simulink model "cic"  (Simulink 6.6)
settings: Solver=VariableStepDiscrete  SolverMode=SingleTasking  StartTime=0.0  StopTime=32768/12.8e6  RelTol=1e-3
PreLoadFcn:
  | load_downconverter_input
undefined symbols (not defined in the file): dfilt
libraries: xbsIndex_r4 x66, dsparch4 x3, dspsigops x2
(part 2 of 2)

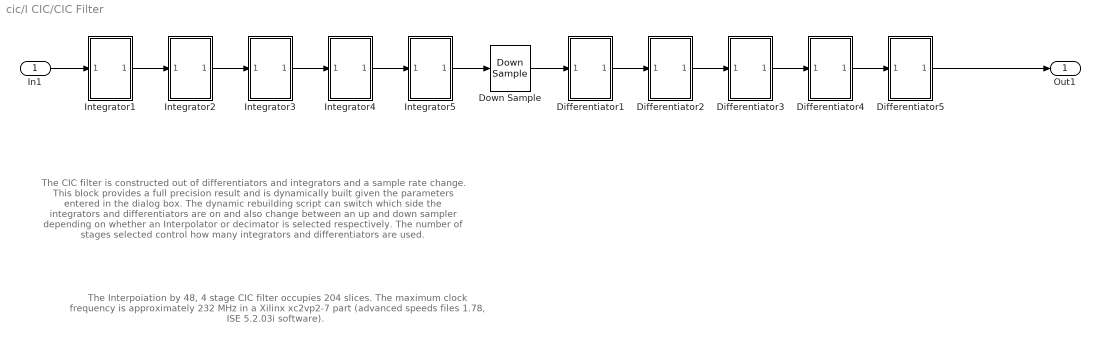
== system cic/I CIC/CIC Filter ==
  note: The Interpoiation by 48, 4 stage CIC filter occupies 204 slices.
      | The maximum clock frequency is approximately
      | 232 MHz in a Xilinx xc2vp2-7 part (advanced speeds
      | files 1.78, ISE 5.2.03i software).
  note: The CIC filter is constructed out of differentiators and integrators and
      | a sample rate change. This block provides a full precision result and is
      | dynamically built given the parameters entered in the dialog box. The
      | dynamic rebuilding script can switch which side the integrators and
      | differentiators are on and also change between an up and down sampler
      | depending on whether an Interpolator or decimator is selected respectively.
      | The number of stages selected control how many integrators and
      | differentiators are used.
  In1 : Inport
  Differentiator1 : Subsystem  mask(Differentiator Stage){m=m, output_bitwidth=ceil(stages*log2(rate_change*m) + input_bitwidth), output_binpt=input_binpt}
      mask prompts: m "Differential Delay"; output_bitwidth "Output Bit Width"; output_binpt "Output Binary Point"
      mask help: Multi-Channel Differentiator
      mask init:
      | set_param(gcb, 'LinkStatus', 'none');
  Differentiator2 : Subsystem  mask(Differentiator Stage){m=m, output_bitwidth=ceil(stages*log2(rate_change*m) + input_bitwidth), output_binpt=input_binpt}
      mask prompts: m "Differential Delay"; output_bitwidth "Output Bit Width"; output_binpt "Output Binary Point"
      mask help: Multi-Channel Differentiator
      mask init:
      | set_param(gcb, 'LinkStatus', 'none');
  Differentiator3 : Subsystem  mask(Differentiator Stage){m=m, output_bitwidth=ceil(stages*log2(rate_change*m) + input_bitwidth), output_binpt=input_binpt}
      mask prompts: m "Differential Delay"; output_bitwidth "Output Bit Width"; output_binpt "Output Binary Point"
      mask help: Multi-Channel Differentiator
      mask init:
      | set_param(gcb, 'LinkStatus', 'none');
  Differentiator4 : Subsystem  mask(Differentiator Stage){m=m, output_bitwidth=ceil(stages*log2(rate_change*m) + input_bitwidth), output_binpt=input_binpt}
      mask prompts: m "Differential Delay"; output_bitwidth "Output Bit Width"; output_binpt "Output Binary Point"
      mask help: Multi-Channel Differentiator
      mask init:
      | set_param(gcb, 'LinkStatus', 'none');
  Differentiator5 : Subsystem  mask(Differentiator Stage){m=m, output_bitwidth=ceil(stages*log2(rate_change*m) + input_bitwidth), output_binpt=input_binpt}
      mask prompts: m "Differential Delay"; output_bitwidth "Output Bit Width"; output_binpt "Output Binary Point"
      mask help: Multi-Channel Differentiator
      mask init:
      | set_param(gcb, 'LinkStatus', 'none');
  Down Sample : xbsIndex_r4/Down Sample  sample_ratio=rate_change  sample_phase=First Value of Frame  en=off  latency=1  dbl_ovrd=off  block_type=dsamp
      settings: block_version=VER_STRING_GOES_HERE
  Integrator1 : Subsystem  mask(Integrator Stage){output_bitwidth=ceil(stages*log2(rate_change*m) + input_bitwidth)}
      mask prompts: output_bitwidth "Output Bit Width"
      mask help: Multi Channel Integrator
      mask init:
      | set_param(gcb, 'LinkStatus', 'none');
      settings: CopyFcn=set_param(gcb, 'LinkStatus', 'none');
  Integrator2 : Subsystem  mask(Integrator Stage){output_bitwidth=ceil(stages*log2(rate_change*m) + input_bitwidth)}
      mask prompts: output_bitwidth "Output Bit Width"
      mask help: Multi Channel Integrator
      mask init:
      | set_param(gcb, 'LinkStatus', 'none');
      settings: CopyFcn=set_param(gcb, 'LinkStatus', 'none');
  Integrator3 : Subsystem  mask(Integrator Stage){output_bitwidth=ceil(stages*log2(rate_change*m) + input_bitwidth)}
      mask prompts: output_bitwidth "Output Bit Width"
      mask help: Multi Channel Integrator
      mask init:
      | set_param(gcb, 'LinkStatus', 'none');
      settings: CopyFcn=set_param(gcb, 'LinkStatus', 'none');
  Integrator4 : Subsystem  mask(Integrator Stage){output_bitwidth=ceil(stages*log2(rate_change*m) + input_bitwidth)}
      mask prompts: output_bitwidth "Output Bit Width"
      mask help: Multi Channel Integrator
      mask init:
      | set_param(gcb, 'LinkStatus', 'none');
      settings: CopyFcn=set_param(gcb, 'LinkStatus', 'none');
  Integrator5 : Subsystem  mask(Integrator Stage){output_bitwidth=ceil(stages*log2(rate_change*m) + input_bitwidth)}
      mask prompts: output_bitwidth "Output Bit Width"
      mask help: Multi Channel Integrator
      mask init:
      | set_param(gcb, 'LinkStatus', 'none');
      settings: CopyFcn=set_param(gcb, 'LinkStatus', 'none');
  Out1 : Outport
  wires:
  In1/1 -> Integrator1/1(In1)
  Down Sample/1 -> Differentiator1/1(In1)
  Integrator1/1(Out1) -> Integrator2/1(In1)
  Differentiator1/1(Out1) -> Differentiator2/1(In1)
  Integrator2/1(Out1) -> Integrator3/1(In1)
  Differentiator2/1(Out1) -> Differentiator3/1(In1)
  Integrator3/1(Out1) -> Integrator4/1(In1)
  Differentiator3/1(Out1) -> Differentiator4/1(In1)
  Integrator4/1(Out1) -> Integrator5/1(In1)
  Differentiator4/1(Out1) -> Differentiator5/1(In1)
  Integrator5/1(Out1) -> Down Sample/1
  Differentiator5/1(Out1) -> Out1/1

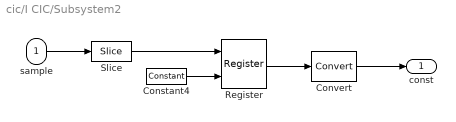
== system cic/I CIC/Subsystem2 ==
  sample : Inport
  Constant4 : xbsIndex_r4/Constant  arith_type=Boolean  const=0  n_bits=1  bin_pt=0  explicit_period=off  period=1  equ=P=C  opselect=C  inp2=PCIN>>17  opr=+  inp1=P  carry=CIN  dbl_ovrd=off  block_type=constant
      settings: block_version=VER_STRING_GOES_HERE
  Convert : xbsIndex_r4/Convert  arith_type=Boolean  n_bits=16  bin_pt=14  quantization=Truncate  overflow=Wrap  latency=0  dbl_ovrd=off  pipeline=off  block_type=convert
      settings: block_version=VER_STRING_GOES_HERE
  Register : xbsIndex_r4/Register  init=1  rst=off  en=on  dbl_ovrd=off  block_type=register
      settings: block_version=VER_STRING_GOES_HERE
  Slice : xbsIndex_r4/Slice  nbits=1  boolean_output=off  mode=Upper Bit Location + Width  bit1=0  base1=MSB of Input  bit0=0  base0=LSB of Input  dbl_ovrd=off  block_type=slice
      settings: infoedit="Extracts a given range of bits from each input sample and presents it at the output.  The output type is ordinarily unsigned with binary point at zero, but can be Boolean when the slice is one bit wide.<P><P>Hardware notes: In hardware this block costs nothing."  block_version=VER_STRING_GOES_HERE
  const : Outport
  wires:
  Constant4/1 -> Register/2
  Slice/1 -> Register/1
  sample/1 -> Slice/1
  Register/1 -> Convert/1
  Convert/1 -> const/1

== system cic/I baseband/I source ==
  Random Number2 : RandomNumber  Seed=777  SampleTime=1/100e3
  Sign2 : Signum
  Out1 : Outport
  wires:
  Random Number2/1 -> Sign2/1
  Sign2/1 -> Out1/1

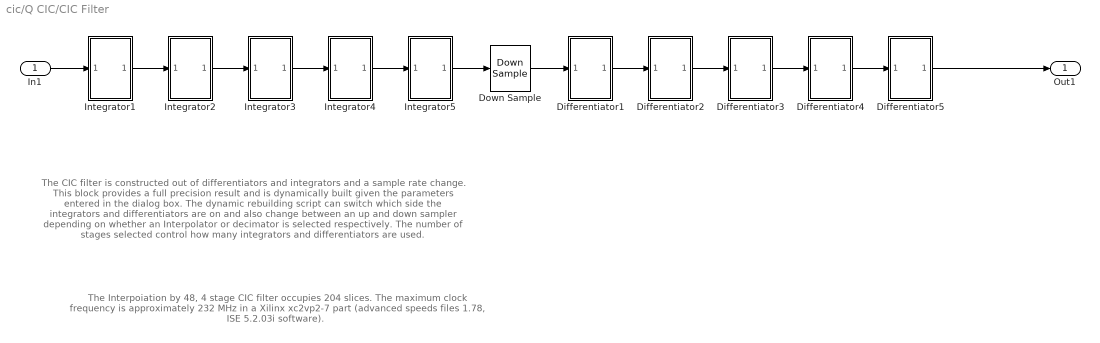
== system cic/Q CIC/CIC Filter ==
  note: The Interpoiation by 48, 4 stage CIC filter occupies 204 slices.
      | The maximum clock frequency is approximately
      | 232 MHz in a Xilinx xc2vp2-7 part (advanced speeds
      | files 1.78, ISE 5.2.03i software).
  note: The CIC filter is constructed out of differentiators and integrators and
      | a sample rate change. This block provides a full precision result and is
      | dynamically built given the parameters entered in the dialog box. The
      | dynamic rebuilding script can switch which side the integrators and
      | differentiators are on and also change between an up and down sampler
      | depending on whether an Interpolator or decimator is selected respectively.
      | The number of stages selected control how many integrators and
      | differentiators are used.
  In1 : Inport
  Differentiator1 : Subsystem  mask(Differentiator Stage){m=m, output_bitwidth=ceil(stages*log2(rate_change*m) + input_bitwidth), output_binpt=input_binpt}
      mask prompts: m "Differential Delay"; output_bitwidth "Output Bit Width"; output_binpt "Output Binary Point"
      mask help: Multi-Channel Differentiator
      mask init:
      | set_param(gcb, 'LinkStatus', 'none');
  Differentiator2 : Subsystem  mask(Differentiator Stage){m=m, output_bitwidth=ceil(stages*log2(rate_change*m) + input_bitwidth), output_binpt=input_binpt}
      mask prompts: m "Differential Delay"; output_bitwidth "Output Bit Width"; output_binpt "Output Binary Point"
      mask help: Multi-Channel Differentiator
      mask init:
      | set_param(gcb, 'LinkStatus', 'none');
  Differentiator3 : Subsystem  mask(Differentiator Stage){m=m, output_bitwidth=ceil(stages*log2(rate_change*m) + input_bitwidth), output_binpt=input_binpt}
      mask prompts: m "Differential Delay"; output_bitwidth "Output Bit Width"; output_binpt "Output Binary Point"
      mask help: Multi-Channel Differentiator
      mask init:
      | set_param(gcb, 'LinkStatus', 'none');
  Differentiator4 : Subsystem  mask(Differentiator Stage){m=m, output_bitwidth=ceil(stages*log2(rate_change*m) + input_bitwidth), output_binpt=input_binpt}
      mask prompts: m "Differential Delay"; output_bitwidth "Output Bit Width"; output_binpt "Output Binary Point"
      mask help: Multi-Channel Differentiator
      mask init:
      | set_param(gcb, 'LinkStatus', 'none');
  Differentiator5 : Subsystem  mask(Differentiator Stage){m=m, output_bitwidth=ceil(stages*log2(rate_change*m) + input_bitwidth), output_binpt=input_binpt}
      mask prompts: m "Differential Delay"; output_bitwidth "Output Bit Width"; output_binpt "Output Binary Point"
      mask help: Multi-Channel Differentiator
      mask init:
      | set_param(gcb, 'LinkStatus', 'none');
  Down Sample : xbsIndex_r4/Down Sample  sample_ratio=rate_change  sample_phase=First Value of Frame  en=off  latency=1  dbl_ovrd=off  block_type=dsamp
      settings: block_version=VER_STRING_GOES_HERE
  Integrator1 : Subsystem  mask(Integrator Stage){output_bitwidth=ceil(stages*log2(rate_change*m) + input_bitwidth)}
      mask prompts: output_bitwidth "Output Bit Width"
      mask help: Multi Channel Integrator
      mask init:
      | set_param(gcb, 'LinkStatus', 'none');
      settings: CopyFcn=set_param(gcb, 'LinkStatus', 'none');
  Integrator2 : Subsystem  mask(Integrator Stage){output_bitwidth=ceil(stages*log2(rate_change*m) + input_bitwidth)}
      mask prompts: output_bitwidth "Output Bit Width"
      mask help: Multi Channel Integrator
      mask init:
      | set_param(gcb, 'LinkStatus', 'none');
      settings: CopyFcn=set_param(gcb, 'LinkStatus', 'none');
  Integrator3 : Subsystem  mask(Integrator Stage){output_bitwidth=ceil(stages*log2(rate_change*m) + input_bitwidth)}
      mask prompts: output_bitwidth "Output Bit Width"
      mask help: Multi Channel Integrator
      mask init:
      | set_param(gcb, 'LinkStatus', 'none');
      settings: CopyFcn=set_param(gcb, 'LinkStatus', 'none');
  Integrator4 : Subsystem  mask(Integrator Stage){output_bitwidth=ceil(stages*log2(rate_change*m) + input_bitwidth)}
      mask prompts: output_bitwidth "Output Bit Width"
      mask help: Multi Channel Integrator
      mask init:
      | set_param(gcb, 'LinkStatus', 'none');
      settings: CopyFcn=set_param(gcb, 'LinkStatus', 'none');
  Integrator5 : Subsystem  mask(Integrator Stage){output_bitwidth=ceil(stages*log2(rate_change*m) + input_bitwidth)}
      mask prompts: output_bitwidth "Output Bit Width"
      mask help: Multi Channel Integrator
      mask init:
      | set_param(gcb, 'LinkStatus', 'none');
      settings: CopyFcn=set_param(gcb, 'LinkStatus', 'none');
  Out1 : Outport
  wires:
  In1/1 -> Integrator1/1(In1)
  Down Sample/1 -> Differentiator1/1(In1)
  Integrator1/1(Out1) -> Integrator2/1(In1)
  Differentiator1/1(Out1) -> Differentiator2/1(In1)
  Integrator2/1(Out1) -> Integrator3/1(In1)
  Differentiator2/1(Out1) -> Differentiator3/1(In1)
  Integrator3/1(Out1) -> Integrator4/1(In1)
  Differentiator3/1(Out1) -> Differentiator4/1(In1)
  Integrator4/1(Out1) -> Integrator5/1(In1)
  Differentiator4/1(Out1) -> Differentiator5/1(In1)
  Integrator5/1(Out1) -> Down Sample/1
  Differentiator5/1(Out1) -> Out1/1

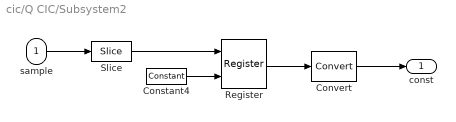
== system cic/Q CIC/Subsystem2 ==
  sample : Inport
  Constant4 : xbsIndex_r4/Constant  arith_type=Boolean  const=0  n_bits=1  bin_pt=0  explicit_period=off  period=1  equ=P=C  opselect=C  inp2=PCIN>>17  opr=+  inp1=P  carry=CIN  dbl_ovrd=off  block_type=constant
      settings: block_version=VER_STRING_GOES_HERE
  Convert : xbsIndex_r4/Convert  arith_type=Boolean  n_bits=16  bin_pt=14  quantization=Truncate  overflow=Wrap  latency=0  dbl_ovrd=off  pipeline=off  block_type=convert
      settings: block_version=VER_STRING_GOES_HERE
  Register : xbsIndex_r4/Register  init=1  rst=off  en=on  dbl_ovrd=off  block_type=register
      settings: block_version=VER_STRING_GOES_HERE
  Slice : xbsIndex_r4/Slice  nbits=1  boolean_output=off  mode=Upper Bit Location + Width  bit1=0  base1=MSB of Input  bit0=0  base0=LSB of Input  dbl_ovrd=off  block_type=slice
      settings: infoedit="Extracts a given range of bits from each input sample and presents it at the output.  The output type is ordinarily unsigned with binary point at zero, but can be Boolean when the slice is one bit wide.<P><P>Hardware notes: In hardware this block costs nothing."  block_version=VER_STRING_GOES_HERE
  const : Outport
  wires:
  Constant4/1 -> Register/2
  Slice/1 -> Register/1
  sample/1 -> Slice/1
  Register/1 -> Convert/1
  Convert/1 -> const/1

== system cic/Q baseband/Q source ==
  Random Number1 : RandomNumber  Seed=99  SampleTime=1/100e3
  Sign1 : Signum
  Out1 : Outport
  wires:
  Random Number1/1 -> Sign1/1
  Sign1/1 -> Out1/1

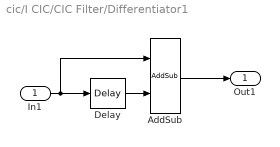
== system cic/I CIC/CIC Filter/Differentiator1 ==
  In1 : Inport
  AddSub : xbsIndex_r4/AddSub  mode=Subtraction  use_carryin=off  use_carryout=off  en=off  latency=1  precision=User Defined  arith_type="Signed  (2's comp)"  n_bits=output_bitwidth  bin_pt=output_binpt  quantization=Truncate  overflow=Wrap  dbl_ovrd=off  use_behavioral_HDL=on  pipelined=off  use_rpm=on  block_type=addsub
      settings: xl_area=[53 106 0 106 0 0 0]  block_version=VER_STRING_GOES_HERE
  Delay : xbsIndex_r4/Delay  en=off  latency=m  dbl_ovrd=off  reg_retiming=off  block_type=delay
      settings: infoedit="Delay line having  configurable length.<P><P>Hardware notes: A delay line is a chain, each link of which is an SRL16 followed by a flip-flop. If register retiming is enabled, the delay line is a chain of flip-flops."  xl_area=[53 106 0 0 0 0 0]  block_version=VER_STRING_GOES_HERE
  Out1 : Outport
  wires:
  Delay/1 -> AddSub/2
  AddSub/1 -> Out1/1
  In1/1 -> AddSub/1, Delay/1

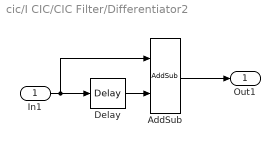
== system cic/I CIC/CIC Filter/Differentiator2 ==
  In1 : Inport
  AddSub : xbsIndex_r4/AddSub  mode=Subtraction  use_carryin=off  use_carryout=off  en=off  latency=1  precision=User Defined  arith_type="Signed  (2's comp)"  n_bits=output_bitwidth  bin_pt=output_binpt  quantization=Truncate  overflow=Wrap  dbl_ovrd=off  use_behavioral_HDL=on  pipelined=off  use_rpm=on  block_type=addsub
      settings: xl_area=[53 106 0 106 0 0 0]  block_version=VER_STRING_GOES_HERE
  Delay : xbsIndex_r4/Delay  en=off  latency=m  dbl_ovrd=off  reg_retiming=off  block_type=delay
      settings: infoedit="Delay line having  configurable length.<P><P>Hardware notes: A delay line is a chain, each link of which is an SRL16 followed by a flip-flop. If register retiming is enabled, the delay line is a chain of flip-flops."  xl_area=[53 106 0 0 0 0 0]  block_version=VER_STRING_GOES_HERE
  Out1 : Outport
  wires:
  In1/1 -> Delay/1, AddSub/1
  AddSub/1 -> Out1/1
  Delay/1 -> AddSub/2

== system cic/I CIC/CIC Filter/Differentiator3 ==
  In1 : Inport
  AddSub : xbsIndex_r4/AddSub  mode=Subtraction  use_carryin=off  use_carryout=off  en=off  latency=1  precision=User Defined  arith_type="Signed  (2's comp)"  n_bits=output_bitwidth  bin_pt=output_binpt  quantization=Truncate  overflow=Wrap  dbl_ovrd=off  use_behavioral_HDL=on  pipelined=off  use_rpm=on  block_type=addsub
      settings: xl_area=[53 106 0 106 0 0 0]  block_version=VER_STRING_GOES_HERE
  Delay : xbsIndex_r4/Delay  en=off  latency=m  dbl_ovrd=off  reg_retiming=off  block_type=delay
      settings: infoedit="Delay line having  configurable length.<P><P>Hardware notes: A delay line is a chain, each link of which is an SRL16 followed by a flip-flop. If register retiming is enabled, the delay line is a chain of flip-flops."  xl_area=[53 106 0 0 0 0 0]  block_version=VER_STRING_GOES_HERE
  Out1 : Outport
  wires:
  In1/1 -> Delay/1, AddSub/1
  AddSub/1 -> Out1/1
  Delay/1 -> AddSub/2

== system cic/I CIC/CIC Filter/Differentiator4 ==
  In1 : Inport
  AddSub : xbsIndex_r4/AddSub  mode=Subtraction  use_carryin=off  use_carryout=off  en=off  latency=1  precision=User Defined  arith_type="Signed  (2's comp)"  n_bits=output_bitwidth  bin_pt=output_binpt  quantization=Truncate  overflow=Wrap  dbl_ovrd=off  use_behavioral_HDL=on  pipelined=off  use_rpm=on  block_type=addsub
      settings: xl_area=[53 106 0 106 0 0 0]  block_version=VER_STRING_GOES_HERE
  Delay : xbsIndex_r4/Delay  en=off  latency=m  dbl_ovrd=off  reg_retiming=off  block_type=delay
      settings: infoedit="Delay line having  configurable length.<P><P>Hardware notes: A delay line is a chain, each link of which is an SRL16 followed by a flip-flop. If register retiming is enabled, the delay line is a chain of flip-flops."  xl_area=[53 106 0 0 0 0 0]  block_version=VER_STRING_GOES_HERE
  Out1 : Outport
  wires:
  In1/1 -> Delay/1, AddSub/1
  AddSub/1 -> Out1/1
  Delay/1 -> AddSub/2

== system cic/I CIC/CIC Filter/Differentiator5 ==
  In1 : Inport
  AddSub : xbsIndex_r4/AddSub  mode=Subtraction  use_carryin=off  use_carryout=off  en=off  latency=1  precision=User Defined  arith_type="Signed  (2's comp)"  n_bits=output_bitwidth  bin_pt=output_binpt  quantization=Truncate  overflow=Wrap  dbl_ovrd=off  use_behavioral_HDL=on  pipelined=off  use_rpm=on  block_type=addsub
      settings: xl_area=[53 106 0 106 0 0 0]  block_version=VER_STRING_GOES_HERE
  Delay : xbsIndex_r4/Delay  en=off  latency=m  dbl_ovrd=off  reg_retiming=off  block_type=delay
      settings: infoedit="Delay line having  configurable length.<P><P>Hardware notes: A delay line is a chain, each link of which is an SRL16 followed by a flip-flop. If register retiming is enabled, the delay line is a chain of flip-flops."  xl_area=[53 106 0 0 0 0 0]  block_version=VER_STRING_GOES_HERE
  Out1 : Outport
  wires:
  In1/1 -> Delay/1, AddSub/1
  AddSub/1 -> Out1/1
  Delay/1 -> AddSub/2

== system cic/I CIC/CIC Filter/Integrator1 ==
  In1 : Inport
  Accumulator : xbsIndex_r4/Accumulator  operation=Add  n_bits=output_bitwidth  overflow=Wrap  scale=1  rst=off  hasbypass=off  en=off  dbl_ovrd=off  use_behavioral_HDL=on  block_type=accum
      settings: infoedit="Adder or subtractor-based accumulator.   Output type and binary point position match the input.<P><P>Hardware notes: When \"Reinitialize with Input 'b' on Reset\" is selected, the accumulator is forced to run at the system rate even if the input 'b' is running at a slower rate."  xl_area=[53 106 0 106 0 0 0]  block_version=VER_STRING_GOES_HERE
  Out1 : Outport
  wires:
  Accumulator/1 -> Out1/1
  In1/1 -> Accumulator/1

== system cic/I CIC/CIC Filter/Integrator2 ==
  In1 : Inport
  Accumulator : xbsIndex_r4/Accumulator  operation=Add  n_bits=output_bitwidth  overflow=Wrap  scale=1  rst=off  hasbypass=off  en=off  dbl_ovrd=off  use_behavioral_HDL=on  block_type=accum
      settings: infoedit="Adder or subtractor-based accumulator.   Output type and binary point position match the input.<P><P>Hardware notes: When \"Reinitialize with Input 'b' on Reset\" is selected, the accumulator is forced to run at the system rate even if the input 'b' is running at a slower rate."  xl_area=[53 106 0 106 0 0 0]  block_version=VER_STRING_GOES_HERE
  Out1 : Outport
  wires:
  In1/1 -> Accumulator/1
  Accumulator/1 -> Out1/1

== system cic/I CIC/CIC Filter/Integrator3 ==
  In1 : Inport
  Accumulator : xbsIndex_r4/Accumulator  operation=Add  n_bits=output_bitwidth  overflow=Wrap  scale=1  rst=off  hasbypass=off  en=off  dbl_ovrd=off  use_behavioral_HDL=on  block_type=accum
      settings: infoedit="Adder or subtractor-based accumulator.   Output type and binary point position match the input.<P><P>Hardware notes: When \"Reinitialize with Input 'b' on Reset\" is selected, the accumulator is forced to run at the system rate even if the input 'b' is running at a slower rate."  xl_area=[53 106 0 106 0 0 0]  block_version=VER_STRING_GOES_HERE
  Out1 : Outport
  wires:
  In1/1 -> Accumulator/1
  Accumulator/1 -> Out1/1

== system cic/I CIC/CIC Filter/Integrator4 ==
  In1 : Inport
  Accumulator : xbsIndex_r4/Accumulator  operation=Add  n_bits=output_bitwidth  overflow=Wrap  scale=1  rst=off  hasbypass=off  en=off  dbl_ovrd=off  use_behavioral_HDL=on  block_type=accum
      settings: infoedit="Adder or subtractor-based accumulator.   Output type and binary point position match the input.<P><P>Hardware notes: When \"Reinitialize with Input 'b' on Reset\" is selected, the accumulator is forced to run at the system rate even if the input 'b' is running at a slower rate."  xl_area=[53 106 0 106 0 0 0]  block_version=VER_STRING_GOES_HERE
  Out1 : Outport
  wires:
  In1/1 -> Accumulator/1
  Accumulator/1 -> Out1/1

== system cic/I CIC/CIC Filter/Integrator5 ==
  In1 : Inport
  Accumulator : xbsIndex_r4/Accumulator  operation=Add  n_bits=output_bitwidth  overflow=Wrap  scale=1  rst=off  hasbypass=off  en=off  dbl_ovrd=off  use_behavioral_HDL=on  block_type=accum
      settings: infoedit="Adder or subtractor-based accumulator.   Output type and binary point position match the input.<P><P>Hardware notes: When \"Reinitialize with Input 'b' on Reset\" is selected, the accumulator is forced to run at the system rate even if the input 'b' is running at a slower rate."  xl_area=[53 106 0 106 0 0 0]  block_version=VER_STRING_GOES_HERE
  Out1 : Outport
  wires:
  In1/1 -> Accumulator/1
  Accumulator/1 -> Out1/1

== system cic/Q CIC/CIC Filter/Differentiator1 ==
  In1 : Inport
  AddSub : xbsIndex_r4/AddSub  mode=Subtraction  use_carryin=off  use_carryout=off  en=off  latency=1  precision=User Defined  arith_type="Signed  (2's comp)"  n_bits=output_bitwidth  bin_pt=output_binpt  quantization=Truncate  overflow=Wrap  dbl_ovrd=off  use_behavioral_HDL=on  pipelined=off  use_rpm=on  block_type=addsub
      settings: xl_area=[53 106 0 106 0 0 0]  block_version=VER_STRING_GOES_HERE
  Delay : xbsIndex_r4/Delay  en=off  latency=m  dbl_ovrd=off  reg_retiming=off  block_type=delay
      settings: infoedit="Delay line having  configurable length.<P><P>Hardware notes: A delay line is a chain, each link of which is an SRL16 followed by a flip-flop. If register retiming is enabled, the delay line is a chain of flip-flops."  xl_area=[53 106 0 0 0 0 0]  block_version=VER_STRING_GOES_HERE
  Out1 : Outport
  wires:
  Delay/1 -> AddSub/2
  AddSub/1 -> Out1/1
  In1/1 -> AddSub/1, Delay/1

== system cic/Q CIC/CIC Filter/Differentiator2 ==
  In1 : Inport
  AddSub : xbsIndex_r4/AddSub  mode=Subtraction  use_carryin=off  use_carryout=off  en=off  latency=1  precision=User Defined  arith_type="Signed  (2's comp)"  n_bits=output_bitwidth  bin_pt=output_binpt  quantization=Truncate  overflow=Wrap  dbl_ovrd=off  use_behavioral_HDL=on  pipelined=off  use_rpm=on  block_type=addsub
      settings: xl_area=[53 106 0 106 0 0 0]  block_version=VER_STRING_GOES_HERE
  Delay : xbsIndex_r4/Delay  en=off  latency=m  dbl_ovrd=off  reg_retiming=off  block_type=delay
      settings: infoedit="Delay line having  configurable length.<P><P>Hardware notes: A delay line is a chain, each link of which is an SRL16 followed by a flip-flop. If register retiming is enabled, the delay line is a chain of flip-flops."  xl_area=[53 106 0 0 0 0 0]  block_version=VER_STRING_GOES_HERE
  Out1 : Outport
  wires:
  In1/1 -> Delay/1, AddSub/1
  AddSub/1 -> Out1/1
  Delay/1 -> AddSub/2

== system cic/Q CIC/CIC Filter/Differentiator3 ==
  In1 : Inport
  AddSub : xbsIndex_r4/AddSub  mode=Subtraction  use_carryin=off  use_carryout=off  en=off  latency=1  precision=User Defined  arith_type="Signed  (2's comp)"  n_bits=output_bitwidth  bin_pt=output_binpt  quantization=Truncate  overflow=Wrap  dbl_ovrd=off  use_behavioral_HDL=on  pipelined=off  use_rpm=on  block_type=addsub
      settings: xl_area=[53 106 0 106 0 0 0]  block_version=VER_STRING_GOES_HERE
  Delay : xbsIndex_r4/Delay  en=off  latency=m  dbl_ovrd=off  reg_retiming=off  block_type=delay
      settings: infoedit="Delay line having  configurable length.<P><P>Hardware notes: A delay line is a chain, each link of which is an SRL16 followed by a flip-flop. If register retiming is enabled, the delay line is a chain of flip-flops."  xl_area=[53 106 0 0 0 0 0]  block_version=VER_STRING_GOES_HERE
  Out1 : Outport
  wires:
  In1/1 -> Delay/1, AddSub/1
  AddSub/1 -> Out1/1
  Delay/1 -> AddSub/2

== system cic/Q CIC/CIC Filter/Differentiator4 ==
  In1 : Inport
  AddSub : xbsIndex_r4/AddSub  mode=Subtraction  use_carryin=off  use_carryout=off  en=off  latency=1  precision=User Defined  arith_type="Signed  (2's comp)"  n_bits=output_bitwidth  bin_pt=output_binpt  quantization=Truncate  overflow=Wrap  dbl_ovrd=off  use_behavioral_HDL=on  pipelined=off  use_rpm=on  block_type=addsub
      settings: xl_area=[53 106 0 106 0 0 0]  block_version=VER_STRING_GOES_HERE
  Delay : xbsIndex_r4/Delay  en=off  latency=m  dbl_ovrd=off  reg_retiming=off  block_type=delay
      settings: infoedit="Delay line having  configurable length.<P><P>Hardware notes: A delay line is a chain, each link of which is an SRL16 followed by a flip-flop. If register retiming is enabled, the delay line is a chain of flip-flops."  xl_area=[53 106 0 0 0 0 0]  block_version=VER_STRING_GOES_HERE
  Out1 : Outport
  wires:
  In1/1 -> Delay/1, AddSub/1
  AddSub/1 -> Out1/1
  Delay/1 -> AddSub/2

== system cic/Q CIC/CIC Filter/Differentiator5 ==
  In1 : Inport
  AddSub : xbsIndex_r4/AddSub  mode=Subtraction  use_carryin=off  use_carryout=off  en=off  latency=1  precision=User Defined  arith_type="Signed  (2's comp)"  n_bits=output_bitwidth  bin_pt=output_binpt  quantization=Truncate  overflow=Wrap  dbl_ovrd=off  use_behavioral_HDL=on  pipelined=off  use_rpm=on  block_type=addsub
      settings: xl_area=[53 106 0 106 0 0 0]  block_version=VER_STRING_GOES_HERE
  Delay : xbsIndex_r4/Delay  en=off  latency=m  dbl_ovrd=off  reg_retiming=off  block_type=delay
      settings: infoedit="Delay line having  configurable length.<P><P>Hardware notes: A delay line is a chain, each link of which is an SRL16 followed by a flip-flop. If register retiming is enabled, the delay line is a chain of flip-flops."  xl_area=[53 106 0 0 0 0 0]  block_version=VER_STRING_GOES_HERE
  Out1 : Outport
  wires:
  In1/1 -> Delay/1, AddSub/1
  AddSub/1 -> Out1/1
  Delay/1 -> AddSub/2

== system cic/Q CIC/CIC Filter/Integrator1 ==
  In1 : Inport
  Accumulator : xbsIndex_r4/Accumulator  operation=Add  n_bits=output_bitwidth  overflow=Wrap  scale=1  rst=off  hasbypass=off  en=off  dbl_ovrd=off  use_behavioral_HDL=on  block_type=accum
      settings: infoedit="Adder or subtractor-based accumulator.   Output type and binary point position match the input.<P><P>Hardware notes: When \"Reinitialize with Input 'b' on Reset\" is selected, the accumulator is forced to run at the system rate even if the input 'b' is running at a slower rate."  xl_area=[53 106 0 106 0 0 0]  block_version=VER_STRING_GOES_HERE
  Out1 : Outport
  wires:
  Accumulator/1 -> Out1/1
  In1/1 -> Accumulator/1

== system cic/Q CIC/CIC Filter/Integrator2 ==
  In1 : Inport
  Accumulator : xbsIndex_r4/Accumulator  operation=Add  n_bits=output_bitwidth  overflow=Wrap  scale=1  rst=off  hasbypass=off  en=off  dbl_ovrd=off  use_behavioral_HDL=on  block_type=accum
      settings: infoedit="Adder or subtractor-based accumulator.   Output type and binary point position match the input.<P><P>Hardware notes: When \"Reinitialize with Input 'b' on Reset\" is selected, the accumulator is forced to run at the system rate even if the input 'b' is running at a slower rate."  xl_area=[53 106 0 106 0 0 0]  block_version=VER_STRING_GOES_HERE
  Out1 : Outport
  wires:
  In1/1 -> Accumulator/1
  Accumulator/1 -> Out1/1

== system cic/Q CIC/CIC Filter/Integrator3 ==
  In1 : Inport
  Accumulator : xbsIndex_r4/Accumulator  operation=Add  n_bits=output_bitwidth  overflow=Wrap  scale=1  rst=off  hasbypass=off  en=off  dbl_ovrd=off  use_behavioral_HDL=on  block_type=accum
      settings: infoedit="Adder or subtractor-based accumulator.   Output type and binary point position match the input.<P><P>Hardware notes: When \"Reinitialize with Input 'b' on Reset\" is selected, the accumulator is forced to run at the system rate even if the input 'b' is running at a slower rate."  xl_area=[53 106 0 106 0 0 0]  block_version=VER_STRING_GOES_HERE
  Out1 : Outport
  wires:
  In1/1 -> Accumulator/1
  Accumulator/1 -> Out1/1

== system cic/Q CIC/CIC Filter/Integrator4 ==
  In1 : Inport
  Accumulator : xbsIndex_r4/Accumulator  operation=Add  n_bits=output_bitwidth  overflow=Wrap  scale=1  rst=off  hasbypass=off  en=off  dbl_ovrd=off  use_behavioral_HDL=on  block_type=accum
      settings: infoedit="Adder or subtractor-based accumulator.   Output type and binary point position match the input.<P><P>Hardware notes: When \"Reinitialize with Input 'b' on Reset\" is selected, the accumulator is forced to run at the system rate even if the input 'b' is running at a slower rate."  xl_area=[53 106 0 106 0 0 0]  block_version=VER_STRING_GOES_HERE
  Out1 : Outport
  wires:
  In1/1 -> Accumulator/1
  Accumulator/1 -> Out1/1

== system cic/Q CIC/CIC Filter/Integrator5 ==
  In1 : Inport
  Accumulator : xbsIndex_r4/Accumulator  operation=Add  n_bits=output_bitwidth  overflow=Wrap  scale=1  rst=off  hasbypass=off  en=off  dbl_ovrd=off  use_behavioral_HDL=on  block_type=accum
      settings: infoedit="Adder or subtractor-based accumulator.   Output type and binary point position match the input.<P><P>Hardware notes: When \"Reinitialize with Input 'b' on Reset\" is selected, the accumulator is forced to run at the system rate even if the input 'b' is running at a slower rate."  xl_area=[53 106 0 106 0 0 0]  block_version=VER_STRING_GOES_HERE
  Out1 : Outport
  wires:
  In1/1 -> Accumulator/1
  Accumulator/1 -> Out1/1
